simulink model "sd"  (R2016a)
settings: Solver=ode15s  StartTime=0.0  StopTime=10.0  RelTol=1e-3
libraries: fl_lib x11, nesl_utility x5
settings Model: Creator=EDU Student  LastModifiedBy=EDU Student

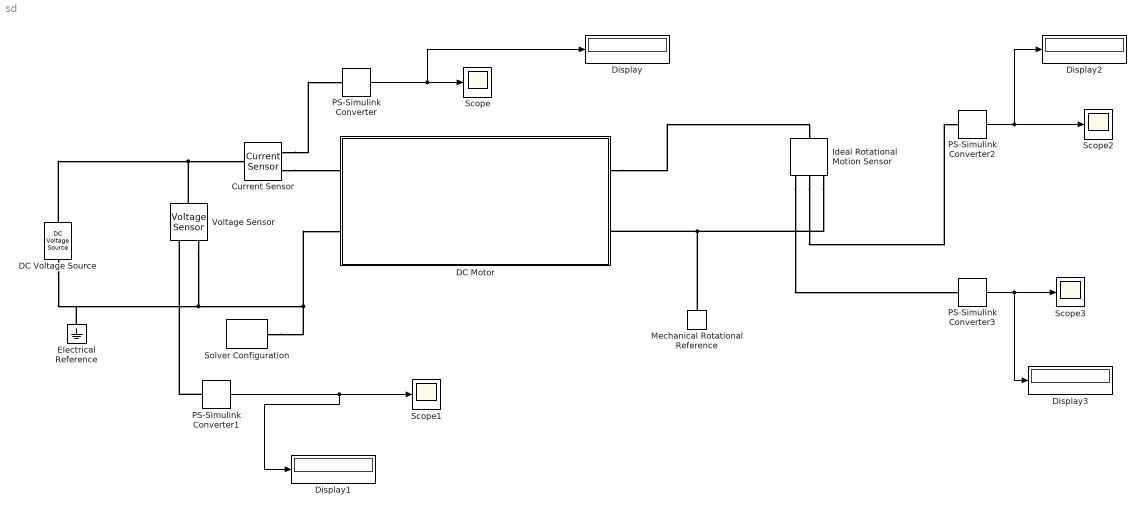
== system sd ==
  Current Sensor : fl_lib/Electrical/Electrical Sensors/Current Sensor
  "DC Motor " : Subsystem
  DC Voltage Source : fl_lib/Electrical/Electrical Sources/DC Voltage Source  v0=220 V
  Display{,1..3} (4 alike) : Display
  Electrical Reference : fl_lib/Electrical/Electrical Elements/Electrical Reference
  Ideal Rotational Motion Sensor : fl_lib/Mechanical/Mechanical Sensors/Ideal Rotational Motion Sensor  offset=0 rad
  Mechanical Rotational Reference : fl_lib/Mechanical/Rotational Elements/Mechanical Rotational Reference
  PS-Simulink Converter{,1..3} (4 alike) : nesl_utility/PS-Simulink Converter  PhysicalDomain=network_engine_domain  SubClassName=ps_output  LeftPortType=input  RightPortType=output  PseudoPeriodic=off  Frequencies=[]  Unit=1  AffineConversion=off
  Scope{,1..3} (4 alike) : Scope
  Solver Configuration : nesl_utility/Solver Configuration  PhysicalDomain=network_engine_domain  SubClassName=solver  LeftPortType=input  RightPortType=generic  Accelerate=off  Tones=[]  Harmonics=[]  SimulateNoise=off  Profile=off  UseLocalSampling=off  EnableSwitchedLinearOptims=on  FrequencyDomain=off  UseCCode=off  RelTol=0.001  AbsTol=1e-06  MinStep=1e-09  ToWorkspace=off  RevertToSquareIcSolve=off  NumHomotopyIterations=100  PhasorMode=off  PhasorModeNumHarmonics=1  OverrideAbsTol=off  DoDC=off  ResidualTolerance=1e-09  UseLocalSolver=off  LocalSolverChoice=NE_BACKWARD_EULER_ADVANCER  LocalSolverSampleTime=0.001  DoFixedCost=off  MaxNonlinIter=3  MaxModeIter=2  LinearAlgebra=Sparse  DelaysMemoryBudget=1024  AutomaticFiltering=on  FilteringTimeConstant=0.001
  Voltage Sensor : fl_lib/Electrical/Electrical Sensors/Voltage Sensor
  wires:
  PS-Simulink Converter/1 -> Display/1, Scope/1
  PS-Simulink Converter1/1 -> Scope1/1, Display1/1
  PS-Simulink Converter2/1 -> Display2/1, Scope2/1
  PS-Simulink Converter3/1 -> Display3/1, Scope3/1
  connections:
  DC Voltage Source/LConn1 -- Voltage Sensor/LConn1 -- Current Sensor/LConn1
  Current Sensor/RConn2 -- "DC Motor "/LConn1
  Voltage Sensor/RConn2 -- Electrical Reference/LConn1 -- DC Voltage Source/RConn1 -- Solver Configuration/RConn1 -- "DC Motor "/LConn2
  "DC Motor "/RConn1 -- Ideal Rotational Motion Sensor/LConn1
  Ideal Rotational Motion Sensor/RConn1 -- Mechanical Rotational Reference/LConn1 -- "DC Motor "/RConn2
  Current Sensor/RConn1 -- PS-Simulink Converter/LConn1
  PS-Simulink Converter1/LConn1 -- Voltage Sensor/RConn1
  Ideal Rotational Motion Sensor/RConn2 -- PS-Simulink Converter2/LConn1
  Ideal Rotational Motion Sensor/RConn3 -- PS-Simulink Converter3/LConn1

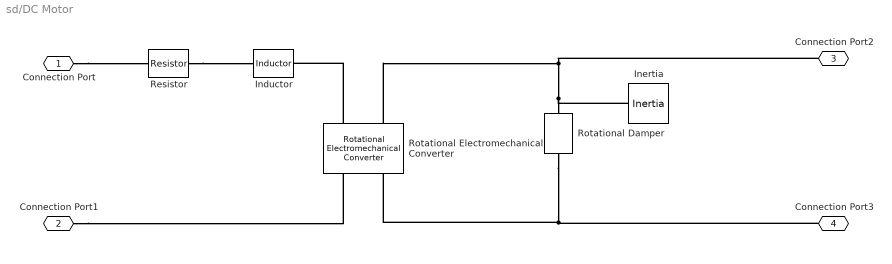
== system sd/DC Motor  ==
  Inductor : fl_lib/Electrical/Electrical Elements/Inductor  l=0.5 H  r=0 Ohm  g=1e-9 1/Ohm  i_specify=off  i_priority=None  i=0 A  v_specify=off  v_priority=None  v=0 V  i_L_specify=off  i_L_priority=High  i_L=0 A
  Inertia : fl_lib/Mechanical/Rotational Elements/Inertia  inertia=0.01 kg*m^2  w_specify=off  w_priority=High  w=0 rad/s  t_specify=off  t_priority=None  t=0 N*m
  Resistor : fl_lib/Electrical/Electrical Elements/Resistor  R=1 Ohm  i_specify=off  i_priority=None  i=0 A  v_specify=off  v_priority=None  v=0 V
  Rotational Electromechanical Converter : fl_lib/Electrical/Electrical Elements/Rotational Electromechanical Converter  K=0.01 V/(rad/s)  i_specify=off  i_priority=None  i=0 A  v_specify=off  v_priority=None  v=0 V  t_specify=off  t_priority=None  t=0 N*m  w_specify=off  w_priority=None  w=0 rad/s
  Rotational Damper : fl_lib/Mechanical/Rotational Elements/Rotational Damper  D=0.1 N*m/(rad/s)  w_specify=off  w_priority=None  w=0 rad/s  t_specify=off  t_priority=None  t=0 N*m
  Connection Port : PMIOPort  Port=1  Side=Left
  Connection Port1 : PMIOPort  Port=2  Side=Left
  Connection Port2 : PMIOPort  Port=3  Side=Right
  Connection Port3 : PMIOPort  Port=4  Side=Right
  connections:
  Rotational Electromechanical Converter/LConn1 -- Inductor/RConn1
  Rotational Electromechanical Converter/LConn2 -- Connection Port2/RConn1 -- Inertia/LConn1 -- Rotational Damper/LConn1
  Resistor/RConn1 -- Inductor/LConn1
  Rotational Damper/RConn1 -- Connection Port3/RConn1 -- Rotational Electromechanical Converter/RConn2
  Connection Port/RConn1 -- Resistor/LConn1
  Connection Port1/RConn1 -- Rotational Electromechanical Converter/RConn1
